simulink model "estimator"  (R2024b)
settings: Solver=FixedStepAuto  StartTime=0.0  StopTime=10.0  FixedStep=0.004  RelTol=1e-3
settings Model: Creator=lukec  LastModifiedBy=lukec

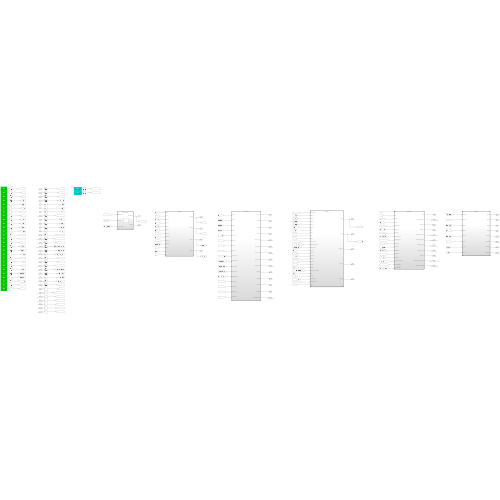
[thumbnail: Simulink's stored preview of the top-level diagram]
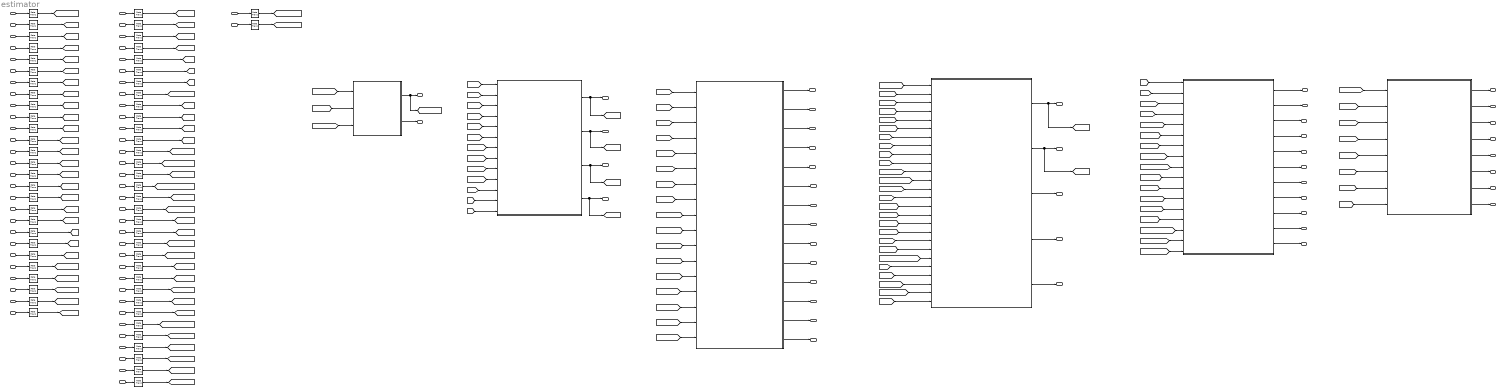
== system estimator ==
  note: non-param-inputs
  note: is-bool
  steer_sensor_raw : Inport
  ax_m_s2 : Inport  Port=2
  ay_m_s2 : Inport  Port=3
  loadcell_fl : Inport  Port=4
  loadcell_fr : Inport  Port=5
  loadcell_rl : Inport  Port=6
  loadcell_rr : Inport  Port=7
  static_fz_N_fl : Inport  Port=8
  static_fz_N_fr : Inport  Port=9
  static_fz_N_rl : Inport  Port=10
  static_fz_N_rr : Inport  Port=11
  cgz_m : Inport  Port=12
  fz_Q : Inport  Port=13
  fz_R : Inport  Port=14
  torq_Nm_fl : Inport  Port=15
  torq_Nm_fr : Inport  Port=16
  torq_Nm_rl : Inport  Port=17
  torq_Nm_rr : Inport  Port=18
  motor_rpm_fl : Inport  Port=19
  motor_rpm_fr : Inport  Port=20
  motor_rpm_rl : Inport  Port=21
  motor_rpm_rr : Inport  Port=22
  amk_eff_modifier_fl : Inport  Port=23
  vx_raw_m_s : Inport  Port=24
  vy_raw_m_s : Inport  Port=25
  vy_Q11 : Inport  Port=26
  wz_Q22 : Inport  Port=27
  vy_R11 : Inport  Port=28
  wz_R22 : Inport  Port=29
  process_noise_vx : Inport  Port=30
  process_noise_yaw_rate : Inport  Port=31
  process_noise_ax : Inport  Port=32
  ins_vel_u : Inport  Port=33
  ins_mode : Inport  Port=34
  accel : Inport  Port=35
  brake : Inport  Port=36
  percent_wheel_diff_noise_gain : Inport  Port=37
  wz_rad_s : Inport  Port=38
  accel_noise_coef : Inport  Port=39
  yaw_rate_noise_coef : Inport  Port=40
  ay_cap_m_s2 : Inport  Port=41
  des_Mz_gain : Inport  Port=42
  drive_motor_torq_lim : Inport  Port=43
  regen_motor_torq_lim : Inport  Port=44
  elec_p_lim_kW : Inport  Port=45
  motor_rpm_lim : Inport  Port=46
  brake_deadzone : Inport  Port=47
  accel_deadzone : Inport  Port=48
  vel_saturation : Inport  Port=49
  per_motor_elec_p_lim_kW : Inport  Port=50
  use_steer_deadzone : Inport  Port=51
  use_intent_w_derate : Inport  Port=52
  amk_eff_modifier_fr : Inport  Port=53
  amk_eff_modifier_rl : Inport  Port=54
  amk_eff_modifier_rr : Inport  Port=55
  global_eff_modifier : Inport  Port=56
  motor_temp_C_fl : Inport  Port=57
  motor_temp_C_fr : Inport  Port=58
  motor_temp_C_rl : Inport  Port=59
  motor_temp_C_rr : Inport  Port=60
  rack_pot_raw : Inport  Port=61
  rack_pot_presence : Inport  Port=62
  Model : ModelReference  ModelNameDialog=wheel_steer_estimator.slx  SimulationMode=Normal  ModelReferenceVersion=1.6
  Model1 : ModelReference  ModelNameDialog=fz_estimator.slx  SimulationMode=Normal  ModelReferenceVersion=1.5
  Model2 : ModelReference  ModelNameDialog=amk_eff_estimator.slx  SimulationMode=Normal  ModelReferenceVersion=1.12
  Model3 : ModelReference  ModelNameDialog=vel_estimator.slx  SimulationMode=Normal  ModelReferenceVersion=1.6
  Model4 : ModelReference  ModelNameDialog=intent_estimator.slx  SimulationMode=Normal  ModelReferenceVersion=1.13
  Model5 : ModelReference  ModelNameDialog=tire_estimator.slx  SimulationMode=Normal  ModelReferenceVersion=1.5
  Rate Transition{,1..61} (62 alike) : RateTransition  OutPortSampleTime=0.004
  wheel_steer_deg : Outport
  fz_est_N_fl : Outport  Port=2
  fz_est_N_fr : Outport  Port=3
  fz_est_N_rl : Outport  Port=4
  fz_est_N_rr : Outport  Port=5
  amk_eff_fl : Outport  Port=6
  amk_eff_fr : Outport  Port=7
  amk_eff_rl : Outport  Port=8
  amk_eff_rr : Outport  Port=9
  amk_elec_p_W_fl : Outport  Port=10
  amk_elec_p_W_fr : Outport  Port=11
  amk_elec_p_W_rl : Outport  Port=12
  amk_elec_p_W_rr : Outport  Port=13
  amk_elec_p_kW_tot : Outport  Port=14
  vx_est_m_s : Outport  Port=15
  vy_est_m_s : Outport  Port=16
  using_front_vel : Outport  Port=17
  ax_est_m_s2 : Outport  Port=18
  wz_est_rad_s : Outport  Port=19
  intent : Outport  Port=20
  max_tot_motor_torq_Nm : Outport  Port=21
  des_wz_rad_s : Outport  Port=22
  des_Mz_Nm : Outport  Port=23
  intent_drive_motor_torq_lim : Outport  Port=24
  intent_regen_motor_torq_lim : Outport  Port=25
  intent_elec_p_lim_kW : Outport  Port=26
  intent_motor_rpm_lim : Outport  Port=27
  kappas_fl : Outport  Port=28
  kappas_fr : Outport  Port=29
  kappas_rl : Outport  Port=30
  kappas_rr : Outport  Port=31
  alpha_deg_fl : Outport  Port=32
  alpha_deg_fr : Outport  Port=33
  alpha_deg_rl : Outport  Port=34
  alpha_deg_rr : Outport  Port=35
  steer_Mz_gain : Outport  Port=36
  intent_per_motor_elec_p_lim_kW : Outport  Port=37
  intent_use_intent_w_derate : Outport  Port=38
  global_eff_fl : Outport  Port=39
  global_eff_fr : Outport  Port=40
  global_eff_rl : Outport  Port=41
  global_eff_rr : Outport  Port=42
  global_elec_p_kW_tot : Outport  Port=43
  rack_pot_flag : Outport  Port=44
  wires:
  steer_sensor_raw/1 -> Rate Transition/1
  [steer_sensor_raw] -> Model/1
  Rate Transition/1 -> [steer_sensor_raw]
  Model/1 -> [wheel_steer_deg], wheel_steer_deg/1
  ax_m_s2/1 -> Rate Transition2/1
  ay_m_s2/1 -> Rate Transition3/1
  [ax_m_s2] -> Model1/1
  [ay_m_s2] -> Model1/2
  loadcell_fl/1 -> Rate Transition4/1
  loadcell_fr/1 -> Rate Transition5/1
  loadcell_rl/1 -> Rate Transition6/1
  loadcell_rr/1 -> Rate Transition7/1
  [loadcell_fl] -> Model1/3
  [loadcell_fr] -> Model1/4
  [loadcell_rl] -> Model1/5
  [loadcell_rr] -> Model1/6
  static_fz_N_fl/1 -> Rate Transition23/1
  static_fz_N_fr/1 -> Rate Transition24/1
  static_fz_N_rl/1 -> Rate Transition35/1
  static_fz_N_rr/1 -> Rate Transition39/1
  [static_fz_N_fl] -> Model1/7
  [static_fz_N_fr] -> Model1/8
  [static_fz_N_rl] -> Model1/9
  [static_fz_N_rr] -> Model1/10
  cgz_m/1 -> Rate Transition40/1
  [cgz_m] -> Model1/11
  fz_Q/1 -> Rate Transition41/1
  fz_R/1 -> Rate Transition42/1
  [fz_Q] -> Model1/12
  [fz_R] -> Model1/13
  Model1/1 -> [fz_est_N_fl], fz_est_N_fl/1
  Model1/2 -> [fz_est_N_fr], fz_est_N_fr/1
  Model1/3 -> [fz_est_N_rl], fz_est_N_rl/1
  Model1/4 -> [fz_est_N_rr], fz_est_N_rr/1
  torq_Nm_fl/1 -> Rate Transition8/1
  torq_Nm_fr/1 -> Rate Transition9/1
  torq_Nm_rl/1 -> Rate Transition10/1
  torq_Nm_rr/1 -> Rate Transition11/1
  motor_rpm_fl/1 -> Rate Transition14/1
  motor_rpm_fr/1 -> Rate Transition15/1
  motor_rpm_rl/1 -> Rate Transition16/1
  motor_rpm_rr/1 -> Rate Transition17/1
  amk_eff_modifier_fl/1 -> Rate Transition43/1
  [torq_Nm_fl] -> Model2/1
  [torq_Nm_fr] -> Model2/2
  [torq_Nm_rl] -> Model2/3
  [torq_Nm_rr] -> Model2/4
  [motor_rpm_fl] -> Model2/5
  [motor_rpm_fr] -> Model2/6
  [motor_rpm_rl] -> Model2/7
  [motor_rpm_rr] -> Model2/8
  [amk_eff_modifier_fl] -> Model2/9
  Model2/1 -> amk_eff_fl/1
  Model2/2 -> amk_eff_fr/1
  Model2/3 -> amk_eff_rl/1
  Model2/4 -> amk_eff_rr/1
  Model2/5 -> amk_elec_p_W_fl/1
  Model2/6 -> amk_elec_p_W_fr/1
  Model2/7 -> amk_elec_p_W_rl/1
  Model2/8 -> amk_elec_p_W_rr/1
  Model2/9 -> amk_elec_p_kW_tot/1
  [wheel_steer_deg] -> Model3/1
  [fz_est_N_fl] -> Model3/2
  [fz_est_N_fr] -> Model3/3
  [fz_est_N_rl] -> Model3/4
  [fz_est_N_rr] -> Model3/5
  vx_raw_m_s/1 -> Rate Transition18/1
  vy_raw_m_s/1 -> Rate Transition19/1
  [vx_raw_m_s] -> Model3/20
  [vy_raw_m_s] -> Model3/6
  vy_Q11/1 -> Rate Transition44/1
  wz_Q22/1 -> Rate Transition45/1
  vy_R11/1 -> Rate Transition25/1
  wz_R22/1 -> Rate Transition26/1
  [vy_Q11] -> Model3/7
  [wz_Q22] -> Model3/8
  [vy_R11] -> Model3/9
  [wz_R22] -> Model3/10
  process_noise_vx/1 -> Rate Transition29/1
  process_noise_yaw_rate/1 -> Rate Transition30/1
  process_noise_ax/1 -> Rate Transition31/1
  ins_vel_u/1 -> Rate Transition12/1
  [process_noise_ax] -> Model3/13
  [process_noise_yaw_rate] -> Model3/12
  [process_noise_vx] -> Model3/11
  [ins_vel_u] -> Model3/14
  [motor_rpm_fl] -> Model3/15
  [motor_rpm_fr] -> Model3/16
  [motor_rpm_rl] -> Model3/17
  [motor_rpm_rr] -> Model3/18
  ins_mode/1 -> Rate Transition13/1
  [ins_mode] -> Model3/19
  accel/1 -> Rate Transition22/1
  brake/1 -> Rate Transition20/1
  percent_wheel_diff_noise_gain/1 -> Rate Transition32/1
  [percent_wheel_diff_noise_gain] -> Model3/21
  [brake] -> Model3/22
  wz_rad_s/1 -> Rate Transition21/1
  [wz_rad_s] -> Model3/23
  [ax_m_s2] -> Model3/26
  accel_noise_coef/1 -> Rate Transition33/1
  yaw_rate_noise_coef/1 -> Rate Transition34/1
  [accel_noise_coef] -> Model3/24
  [yaw_rate_noise_coef] -> Model3/25
  Model3/1 -> [vx_est_m_s], vx_est_m_s/1
  Model3/2 -> [vy_est_m_s], vy_est_m_s/1
  Model3/3 -> using_front_vel/1
  Model3/4 -> ax_est_m_s2/1
  Model3/5 -> wz_est_rad_s/1
  [accel] -> Model4/1
  [brake] -> Model4/2
  [vx_est_m_s] -> Model4/3
  [wz_rad_s] -> Model4/4
  [wheel_steer_deg] -> Model4/5
  ay_cap_m_s2/1 -> Rate Transition27/1
  des_Mz_gain/1 -> Rate Transition28/1
  [ay_cap_m_s2] -> Model4/6
  [des_Mz_gain] -> Model4/7
  drive_motor_torq_lim/1 -> Rate Transition38/1
  regen_motor_torq_lim/1 -> Rate Transition36/1
  [drive_motor_torq_lim] -> Model4/8
  [regen_motor_torq_lim] -> Model4/9
  elec_p_lim_kW/1 -> Rate Transition37/1
  motor_rpm_lim/1 -> Rate Transition48/1
  brake_deadzone/1 -> Rate Transition46/1
  accel_deadzone/1 -> Rate Transition47/1
  [elec_p_lim_kW] -> Model4/10
  [motor_rpm_lim] -> Model4/11
  [brake_deadzone] -> Model4/12
  [accel_deadzone] -> Model4/13
  Model4/1 -> intent/1
  Model4/2 -> max_tot_motor_torq_Nm/1
  Model4/3 -> des_wz_rad_s/1
  Model4/4 -> des_Mz_Nm/1
  Model4/5 -> intent_drive_motor_torq_lim/1
  Model4/6 -> intent_regen_motor_torq_lim/1
  Model4/7 -> intent_elec_p_lim_kW/1
  Model4/8 -> intent_motor_rpm_lim/1
  [wheel_steer_deg] -> Model5/1
  [motor_rpm_fl] -> Model5/2
  [motor_rpm_fr] -> Model5/3
  [motor_rpm_rl] -> Model5/4
  [motor_rpm_rr] -> Model5/5
  [vx_est_m_s] -> Model5/6
  [vy_est_m_s] -> Model5/7
  [wz_rad_s] -> Model5/8
  Model5/1 -> kappas_fl/1
  Model5/2 -> kappas_fr/1
  Model5/3 -> kappas_rl/1
  Model5/4 -> kappas_rr/1
  Model5/5 -> alpha_deg_fl/1
  Model5/6 -> alpha_deg_fr/1
  Model5/7 -> alpha_deg_rl/1
  Model5/8 -> alpha_deg_rr/1
  Rate Transition2/1 -> [ax_m_s2]
  Rate Transition3/1 -> [ay_m_s2]
  Rate Transition7/1 -> [loadcell_rr]
  Rate Transition4/1 -> [loadcell_fl]
  Rate Transition5/1 -> [loadcell_fr]
  Rate Transition6/1 -> [loadcell_rl]
  Rate Transition9/1 -> [torq_Nm_fr]
  Rate Transition10/1 -> [torq_Nm_rl]
  Rate Transition11/1 -> [torq_Nm_rr]
  Rate Transition8/1 -> [torq_Nm_fl]
  Rate Transition15/1 -> [motor_rpm_fr]
  Rate Transition16/1 -> [motor_rpm_rl]
  Rate Transition17/1 -> [motor_rpm_rr]
  Rate Transition19/1 -> [vy_raw_m_s]
  Rate Transition13/1 -> [ins_mode]
  Rate Transition14/1 -> [motor_rpm_fl]
  Rate Transition18/1 -> [vx_raw_m_s]
  Rate Transition12/1 -> [ins_vel_u]
  Rate Transition21/1 -> [wz_rad_s]
  Rate Transition22/1 -> [accel]
  Rate Transition20/1 -> [brake]
  Rate Transition33/1 -> [accel_noise_coef]
  Rate Transition31/1 -> [process_noise_ax]
  Rate Transition26/1 -> [wz_R22]
  Rate Transition27/1 -> [ay_cap_m_s2]
  Rate Transition24/1 -> [static_fz_N_fr]
  Rate Transition32/1 -> [percent_wheel_diff_noise_gain]
  Rate Transition34/1 -> [yaw_rate_noise_coef]
  Rate Transition25/1 -> [vy_R11]
  Rate Transition28/1 -> [des_Mz_gain]
  Rate Transition35/1 -> [static_fz_N_rl]
  Rate Transition29/1 -> [process_noise_vx]
  Rate Transition30/1 -> [process_noise_yaw_rate]
  Rate Transition38/1 -> [drive_motor_torq_lim]
  Rate Transition37/1 -> [elec_p_lim_kW]
  Rate Transition40/1 -> [cgz_m]
  Rate Transition43/1 -> [amk_eff_modifier_fl]
  Rate Transition39/1 -> [static_fz_N_rr]
  Rate Transition23/1 -> [static_fz_N_fl]
  Rate Transition42/1 -> [fz_R]
  Rate Transition41/1 -> [fz_Q]
  Rate Transition36/1 -> [regen_motor_torq_lim]
  Rate Transition45/1 -> [wz_Q22]
  Rate Transition44/1 -> [vy_Q11]
  Rate Transition47/1 -> [accel_deadzone]
  Rate Transition48/1 -> [motor_rpm_lim]
  Rate Transition46/1 -> [brake_deadzone]
  vel_saturation/1 -> Rate Transition49/1
  Rate Transition49/1 -> [vel_saturation]
  [vel_saturation] -> Model4/14
  Model4/9 -> steer_Mz_gain/1
  Model4/10 -> intent_per_motor_elec_p_lim_kW/1
  per_motor_elec_p_lim_kW/1 -> Rate Transition50/1
  Rate Transition50/1 -> [per_motor_elec_p_lim_kW]
  [per_motor_elec_p_lim_kW] -> Model4/15
  use_steer_deadzone/1 -> Rate Transition51/1
  Rate Transition51/1 -> [use_steer_deadzone]
  [use_steer_deadzone] -> Model4/16
  [use_intent_w_derate] -> Model4/17
  Model4/11 -> intent_use_intent_w_derate/1
  use_intent_w_derate/1 -> Rate Transition52/1
  Rate Transition52/1 -> [use_intent_w_derate]
  amk_eff_modifier_fr/1 -> Rate Transition53/1
  amk_eff_modifier_rl/1 -> Rate Transition54/1
  amk_eff_modifier_rr/1 -> Rate Transition55/1
  Rate Transition54/1 -> [amk_eff_modifier_rl]
  Rate Transition55/1 -> [amk_eff_modifier_rr]
  Rate Transition53/1 -> [amk_eff_modifier_fr]
  [amk_eff_modifier_fr] -> Model2/10
  [amk_eff_modifier_rl] -> Model2/11
  [amk_eff_modifier_rr] -> Model2/12
  global_eff_modifier/1 -> Rate Transition56/1
  Rate Transition56/1 -> [global_eff_modifier]
  [global_eff_modifier] -> Model2/13
  Model2/10 -> global_eff_fl/1
  Model2/11 -> global_eff_fr/1
  Model2/12 -> global_eff_rl/1
  Model2/13 -> global_eff_rr/1
  Model2/14 -> global_elec_p_kW_tot/1
  motor_temp_C_fl/1 -> Rate Transition1/1
  motor_temp_C_fr/1 -> Rate Transition59/1
  motor_temp_C_rl/1 -> Rate Transition57/1
  motor_temp_C_rr/1 -> Rate Transition58/1
  Rate Transition57/1 -> [motor_temp_C_rl]
  Rate Transition58/1 -> [motor_temp_C_rr]
  Rate Transition59/1 -> [motor_temp_C_fr]
  Rate Transition1/1 -> [motor_temp_C_fl]
  [motor_temp_C_fl] -> Model2/14
  [motor_temp_C_fr] -> Model2/15
  [motor_temp_C_rl] -> Model2/16
  [motor_temp_C_rr] -> Model2/17
  rack_pot_raw/1 -> Rate Transition60/1
  Rate Transition60/1 -> [rack_pot_raw]
  rack_pot_presence/1 -> Rate Transition61/1
  Rate Transition61/1 -> [rack_pot_presence]
  [rack_pot_raw] -> Model/2
  [rack_pot_presence] -> Model/3
  Model/2 -> rack_pot_flag/1
